simulink model "smm_with_grf_tilting_2d"  (R2014b)
settings: Solver=FixedStepDiscrete  StartTime=0.0  StopTime=inf  FixedStep=sample_time  RelTol=1e-3
undefined symbols (not defined in the file or in its folder): A_kalman_fourbar_gear, A_kalman_transverse, A_kalman_vertical, A_lpf_dtau, A_lpf_leg_spring, alpha_apex, B1_lpf_dtau, B1_lpf_leg_spring, B2_lpf_dtau, B2_lpf_leg_spring, B_kalman_fourbar_gear, B_kalman_transverse, B_kalman_vertical, b_virtual, boom_mount_angle, c_energy, C_kalman_fourbar_gear, C_kalman_transverse, C_kalman_vertical, com_leg_motor, com_torso, contact_threshold, control_start_time, d_vertical_boom_com_offset, d_vertical_com, d_y_com, desired_com_apex_height, desired_com_forward_velocity, desired_torso_angle, Discrete, fcut_contact, g, h_boom, HIP_MTR_MAX_CONT_TORQUE, i_robot, initial_dx_estimate, initial_dy_estimate, initial_dz_estimate, initial_z_estimate, j_leg, j_motor, j_rotor, j_segments, k0_virtual, k_placement, k_sea, kalman_load_to_deflect_transmission, kalman_stance_slip_threshold, kd_lateral, kd_motor, kd_torso, kp_lateral, kp_motor, kp_torso, l0_leg, l0_virtual, l_boom_projected, l_retract_delta, l_retract_swing_max, l_retract_swing_min ... (+59)
libraries: simulink x25, ctrlSharedLib x7, simulink_extras x1
(part 4 of 4)

== matlab function smm_with_grf_tilting_2d/Control/Behavior Control/Lateral Control ==
  data: hopping input; tau_r output size=1; qLateralR input; dqLateralR input; qLateralL input; dqLateralL input; F_leg_R input; F_leg_L input; lateral_transition_force parameter; lateral_target_angle_right parameter; m_leg_motor parameter; m_leg parameter; m_total_real parameter; g parameter; lateral_offset parameter; tau_l output size=1; kp_lateral parameter; kd_lateral parameter; minimum_lateral_angle parameter; maximum_lateral_angle parameter; HIP_MTR_MAX_CONT_TORQUE parameter; torso_centerline_roll_offset_angle parameter
function [tau_r, tau_l] = LateralBoomControl(hopping, qLateralR, dqLateralR, qLateralL, dqLateralL, F_leg_R, F_leg_L, lateral_transition_force, lateral_target_angle_right, m_leg_motor, m_leg, m_total_real, g, lateral_offset, kp_lateral, kd_lateral, minimum_lateral_angle, maximum_lateral_angle, HIP_MTR_MAX_CONT_TORQUE, torso_centerline_roll_offset_angle)
    
    % Only add gravity compensation to PD when suspended from winch (approximately static)
    gravity_compensation = 0;
    if ~hopping, gravity_compensation = (m_leg_motor+m_leg)*g*lateral_offset; end
    
    % Inertia for feedforward accelerations
    motor_inertia = (m_leg_motor+m_leg)*lateral_offset^2;
    
    % Right Leg
    right_target = [lateral_target_angle_right, 0, 0];
    desired = [saturate(right_target(1),minimum_lateral_angle,maximum_lateral_angle), right_target(2)];
    measured = [qLateralR, dqLateralR];
    tau_r = [kp_lateral, kd_lateral] * (desired-measured)' + gravity_compensation + motor_inertia*right_target(3);
    tau_r = max(min(HIP_MTR_MAX_CONT_TORQUE, tau_r),-HIP_MTR_MAX_CONT_TORQUE);
    
    if (F_leg_R >= lateral_transition_force)
        if hopping
            tau_r = -F_leg_R*lateral_offset*(m_total_real-(m_leg_motor+m_leg))/m_total_real;
        else
            tau_r = -lateral_offset*(F_leg_R-(m_leg_motor+m_leg)*g);
        end
    end
    
    % Left Leg
    left_target = [lateral_target_angle_right, 0, 0];
    desired = [saturate(left_target(1),minimum_lateral_angle,maximum_lateral_angle), left_target(2)];
    measured = [qLateralL, dqLateralL];
    tau_l = [kp_lateral, kd_lateral] * (desired-measured)' + gravity_compensation + motor_inertia*left_target(3);
    tau_l = max(min(HIP_MTR_MAX_CONT_TORQUE, tau_l),-HIP_MTR_MAX_CONT_TORQUE);
    
    if (F_leg_L >= lateral_transition_force)
        if hopping
            tau_l = -F_leg_L*lateral_offset*(m_total_real-(m_leg_motor+m_leg))/m_total_real;
        else
            tau_l = -lateral_offset*(F_leg_L-(m_leg_motor+m_leg)*g);
        end
    end
end

function [desired_saturated] = saturate(desired, minimum_lateral_angle, maximum_lateral_angle)
    desired_saturated = desired;
    if desired(1) < minimum_lateral_angle
        desired_saturated = [minimum_lateral_angle, 0];
    elseif desired(1) > maximum_lateral_angle
        desired_saturated = [maximum_lateral_angle, 0];    
    end
end

== matlab function smm_with_grf_tilting_2d/Control/Behavior Control/Torque Distribution Right/Motor Torque Saturation Optimization ==
  data: x1s input; t1 output; x2s input; lambda1 parameter; lambda2 parameter; max_torque_sagittal parameter; t2 output
% Optimal leg motor torque distribution
function [t1, t2] = distribute_torque(x1s, x2s, lambda1, lambda2, max_torque_sagittal)

s = max_torque_sagittal;

% possible solutions
x1 = [                                                      x1s;
                                                            0;
                                                            s;
                                                            0;
                                                           -s;
  (lambda2*s + lambda1*x1s - lambda2*x2s)/(lambda1 + lambda2);
  (lambda1*x1s - lambda2*s + lambda2*x2s)/(lambda1 + lambda2);
  (lambda2*s + lambda1*x1s + lambda2*x2s)/(lambda1 + lambda2);
 -(lambda2*s - lambda1*x1s + lambda2*x2s)/(lambda1 + lambda2)];
 
x2 = [                                                      x2s;
                                                            s;
                                                            0;
                                                           -s;
                                                            0;
  (lambda1*s - lambda1*x1s + lambda2*x2s)/(lambda1 + lambda2);
  (lambda1*s + lambda1*x1s + lambda2*x2s)/(lambda1 + lambda2);
  (lambda1*x1s - lambda1*s + lambda2*x2s)/(lambda1 + lambda2);
 -(lambda1*s + lambda1*x1s - lambda2*x2s)/(lambda1 + lambda2)];

% test constraints
c1 = s - x1 - x2 >= 0;
c2 = s + x1 + x2 >= 0;
c3 = s - x1 + x2 >= 0;
c4 = s + x1 - x2 >= 0;
constraints = c1 & c2 & c3 & c4;

% objective function to maximize
f = -lambda1*(x1-x1s).^2-lambda2*(x2-x2s).^2;
satisfied = find(constraints);
[~,I] = max(f(satisfied));

t1 = x1(satisfied(I));
t2 = x2(satisfied(I));

== matlab function smm_with_grf_tilting_2d/Control/Behavior Control/Primary Leg Behavior/Running/Flight/Calculate Leg Length From Virtual Spring Length ==
  data: phi input; dphi input; l_virtual input; dl_virtual input; pelvis_to_com input; l_leg_target output; d_pelvis_to_com input
function l_leg_target  = VirtualSpringLengthToLegLength2D(phi, dphi, l_virtual, dl_virtual, pelvis_to_com, d_pelvis_to_com)
    [ l_leg_target, ~ ] = VirtualSpringLengthToLegLength2D( phi, dphi, l_virtual, dl_virtual, pelvis_to_com, d_pelvis_to_com );
end

== matlab function smm_with_grf_tilting_2d/Control/Behavior Control/Secondary Leg Behavior/Avoid Hitting Mechanical Limits ==
  data: back_cmd output double; front_cmd output double; dback_cmd output double; dfront_cmd output double; ddback_cmd output double; ddfront_cmd output double; back_desired input; dback_desired input; ddback_desired input; front_desired input; dfront_desired input; ddfront_desired input; min_front_bar_angle parameter; max_front_bar_angle parameter; min_back_bar_angle parameter; max_back_bar_angle parameter
%% Avoid joint limits by ensuring we don't command velocities/accelerations that would push us into them when we are close to them.
function [back_cmd, front_cmd, dback_cmd, dfront_cmd, ddback_cmd, ddfront_cmd] ...
    = AvoidFourbarLimits(back_desired,dback_desired, ddback_desired, ...
          front_desired, dfront_desired, ddfront_desired, ...
          min_front_bar_angle, max_front_bar_angle, min_back_bar_angle, max_back_bar_angle)
    [back_cmd, front_cmd, dback_cmd, dfront_cmd, ddback_cmd, ddfront_cmd] = AvoidFourbarLimits(back_desired,dback_desired, ddback_desired, front_desired, dfront_desired, ddfront_desired, min_front_bar_angle, max_front_bar_angle, min_back_bar_angle, max_back_bar_angle);
end

== matlab function smm_with_grf_tilting_2d/Control/Behavior Control/State Estimation/PositionUsingRobotGeometry ==
  data: right_left input; horizontal_com_position output; roll input; pitch input; yaw input; horizontal_com_velocity output; left_leg_sagittal_angle input; left_leg_lateral_angle input; left_leg_length input; right_leg_sagittal_angle input; right_leg_lateral_angle input; right_leg_length input; m_torso parameter; m_leg_motor parameter; m_leg parameter; com_torso parameter; com_leg_motor parameter; lateral_offset parameter; vertical_com_position output; vertical_com_velocity output; com_left_foot output; dcom_left_foot output; com_right_foot output; dcom_right_foot output; com_pelvis output; dcom_pelvis output
% Returns 2D COM relative to primary foot
function [horizontal_com_position, horizontal_com_velocity, ...
          vertical_com_position, vertical_com_velocity, ...
          com_left_foot, dcom_left_foot, com_right_foot, dcom_right_foot, ....
          com_pelvis, dcom_pelvis] = ...
         ComPositionUsingRobotGeometry(right_left, ...
                                    roll, pitch, yaw, ...
                                    left_leg_sagittal_angle, left_leg_lateral_angle, left_leg_length, ...
                                    right_leg_sagittal_angle, right_leg_lateral_angle, right_leg_length, ...
                                    m_torso, m_leg_motor, m_leg, com_torso, com_leg_motor, lateral_offset)
                    
    q =  [roll(1), pitch(1), yaw(1), left_leg_sagittal_angle(1), left_leg_lateral_angle(1), left_leg_length(1), right_leg_sagittal_angle(1), right_leg_lateral_angle(1), right_leg_length(1)];
    dq = [roll(2), pitch(2), yaw(2), left_leg_sagittal_angle(2), left_leg_lateral_angle(2), left_leg_length(2), right_leg_sagittal_angle(2), right_leg_lateral_angle(2), right_leg_length(2)];
                    
    [ com_pelvis, dcom_pelvis, ...
      com_left_foot, dcom_left_foot, ...
      com_right_foot, dcom_right_foot ] = ...
    ComCalculationFromRobot( q, dq, m_torso, m_leg_motor, m_leg, com_torso, com_leg_motor, lateral_offset );

    if right_left
        com_position = com_right_foot(4:6);
        com_velocity = dcom_right_foot(4:6);
    else
        com_position = com_left_foot(4:6);
        com_velocity = dcom_left_foot(4:6);
    end


    horizontal_com_position = com_position(1);
    horizontal_com_velocity = com_velocity(1);
    vertical_com_position = com_position(3);
    vertical_com_velocity = com_velocity(3);

end

== matlab function smm_with_grf_tilting_2d/Control/Behavior Control/Torque Distribution Left/Motor Torque Saturation Optimization ==
  data: x1s input; t1 output; x2s input; lambda1 parameter; lambda2 parameter; max_torque_sagittal parameter; t2 output
% Optimal leg motor torque distribution
function [t1, t2] = distribute_torque(x1s, x2s, lambda1, lambda2, max_torque_sagittal)

s = max_torque_sagittal;

% possible solutions
x1 = [                                                      x1s;
                                                            0;
                                                            s;
                                                            0;
                                                           -s;
  (lambda2*s + lambda1*x1s - lambda2*x2s)/(lambda1 + lambda2);
  (lambda1*x1s - lambda2*s + lambda2*x2s)/(lambda1 + lambda2);
  (lambda2*s + lambda1*x1s + lambda2*x2s)/(lambda1 + lambda2);
 -(lambda2*s - lambda1*x1s + lambda2*x2s)/(lambda1 + lambda2)];
 
x2 = [                                                      x2s;
                                                            s;
                                                            0;
                                                           -s;
                                                            0;
  (lambda1*s - lambda1*x1s + lambda2*x2s)/(lambda1 + lambda2);
  (lambda1*s + lambda1*x1s + lambda2*x2s)/(lambda1 + lambda2);
  (lambda1*x1s - lambda1*s + lambda2*x2s)/(lambda1 + lambda2);
 -(lambda1*s + lambda1*x1s - lambda2*x2s)/(lambda1 + lambda2)];

% test constraints
c1 = s - x1 - x2 >= 0;
c2 = s + x1 + x2 >= 0;
c3 = s - x1 + x2 >= 0;
c4 = s + x1 - x2 >= 0;
constraints = c1 & c2 & c3 & c4;

% objective function to maximize
f = -lambda1*(x1-x1s).^2-lambda2*(x2-x2s).^2;
satisfied = find(constraints);
[~,I] = max(f(satisfied));

t1 = x1(satisfied(I));
t2 = x2(satisfied(I));

== matlab function smm_with_grf_tilting_2d/Control/Behavior Control/State Estimation/Kalman Filtering/eigen values ==
  data: Z input; E output
function E = eigen(Z)
    E = real(eig(Z));
    E = sort(E);
end

== matlab function smm_with_grf_tilting_2d/Control/Behavior Control/Virtual Spring Calculator/Virtual Spring Calculations ==
  data: th input; alpha_v output; dth input; l input; dl input; phi input; dphi input; dalpha_v output; l_v output; dl_v output; d_vertical_com parameter
function [alpha_v, dalpha_v, l_v, dl_v] = fcn(th, dth, l, dl, phi, dphi, d_vertical_com)

    gma = th + phi;
    dgma = dth + dphi;
    d = d_vertical_com;

    xf  =  l*sin(gma) - d*sin(th);
    dxf =  l*dgma*cos(gma) + dl*sin(gma) - d*dth*cos(th);
    yf  = -l*cos(gma) + d*cos(th);
    dyf =  l*dgma*sin(gma) - dl*cos(gma) - d*dth*sin(th);

    alpha_v  = atan2(yf, xf);
    dalpha_v = 1/(1+(yf/xf)^2) * (xf*dyf - yf*dxf)/xf^2;

    l_v  = (d^2 + l^2 - 2*d*l*cos(phi))^0.5;
    dl_v = (l*dl - d*dl*cos(phi) + d*l*dphi*sin(phi))/l_v;

end

== matlab function smm_with_grf_tilting_2d/Control/Behavior Control/Secondary Leg Behavior/Virtual Leg Trajectory Towards Alpha Apex Target ==
  data: start input; t_system input; l_leg output; dl_leg output; ddl_leg output; phi output; dphi output; ddphi output; alpha_apex parameter; theta input; l_measured input; dl_measured input; phi_measured input; dphi_measured input; d_y_com parameter; l0_virtual parameter
%% Create a trajectory between starting position/velocity and some alpha
% The goal is to move the system towards the alpha target at apex.
function [l_leg, dl_leg, ddl_leg, phi, dphi, ddphi] = fcn(start, t_system, alpha_apex, theta, l_measured, dl_measured, phi_measured, dphi_measured, d_y_com, l0_virtual)
    % Should the target be less than apex position? midpoint?
    [l_apex, dl_apex, ~, phi_apex, dphi_apex, ~] = AlphaTargetToVirtualLeg2D(alpha_apex, 0, 0, theta, 0, 0, d_y_com, l0_virtual);
    
    % Force retraction when secondary leg
    l_apex = 0.8;
    dl_apex = 0;
    
    persistent t_start l_start phi_start dl_start dphi_start;
    if isempty(t_start)
        t_start = t_system;
        l_start = l_measured;
        dl_start = dl_measured;
        phi_start = phi_measured;
        dphi_start = dphi_measured;
    end
    if start %|| (t_system - t_start) > 0.030
        t_start = t_system;
        l_start = l_measured;
        dl_start = dl_measured;
        phi_start = phi_measured;
        dphi_start = dphi_measured;
    end
    

    time_to_takeoff = 0.350;  % Overestimate, How to approximate this?
    t = t_system - t_start;
    t = min(time_to_takeoff, t);
    
    % Virtual Leg Length
    [a0, a1, a2, a3] = ThirdOrderTrajectory(l_start, dl_start, l_apex, dl_apex, time_to_takeoff);
    l_leg = a3*t^3 + a2*t^2 + a1*t + a0;
    dl_leg = 3*a3*t^2 + 2*a2*t + a1;
    ddl_leg = 6*a3*t + 2*a2;
    
    % Virtual Leg Angle
    [a0, a1, a2, a3] = ThirdOrderTrajectory(phi_start, dphi_start, phi_apex, dphi_apex, time_to_takeoff);
    phi = a3*t^3 + a2*t^2 + a1*t + a0;
    dphi = 3*a3*t^2 + 2*a2*t + a1;
    ddphi = 6*a3*t + 2*a2;
end

== matlab function smm_with_grf_tilting_2d/Control/Behavior Control/Secondary Leg Behavior/Virtual Leg to Four Bar ==
  data: l_leg input; dl_leg input; ddl_leg input; phi input; dphi input; ddphi input; back output; dback output; ddback output; front output; dfront output; ddfront output
function [back, dback, ddback, front, dfront, ddfront] = VirtualLegToFourBar(l_leg, dl_leg, ddl_leg, phi, dphi, ddphi)
    [back, dback, ddback, front, dfront, ddfront] = VirtualLegToFourBar(l_leg, dl_leg, ddl_leg, phi, dphi, ddphi);
end

== matlab function smm_with_grf_tilting_2d/Control/Behavior Control/Primary Secondary Leg Swap/ToggleRightLeftLeg ==
  data: toggle input boolean; right_left output double; previous_right_left input double
function right_left = ToggleRightLeftLeg(toggle, previous_right_left)
    
    if toggle
        right_left = -previous_right_left + 1;
    else
        right_left = previous_right_left;
    end

end

== matlab function smm_with_grf_tilting_2d/Control/Behavior Control/Primary Leg Behavior/Running/Stance/Inverse Dynamics Virtual Spring/target_GRF_inverse_dynamics ==
  data: right_left input; z output; k_virtual input; b_virtual input; l_virtual input; theta input; phi input; l_leg input; w input; tau_rotor_f input; tau_rotor_b input; d_vertical_com parameter; l_virtual_rest input; LEG_MTR_GEAR_RATIO parameter; g parameter; j_leg parameter; j_rotor parameter; i_robot parameter; m_total_real parameter; m_leg parameter; GRFx output; GRFy output; kp_torso parameter; kd_torso parameter; desired_torso_angle input; GRF_angle output; max_GRF_angle parameter
%% Inverse dynamics
% Inputs:  gamma, dgamma, theta, dtheta,  GRFx_des, GRFy_des
% Outputs: ddx,   ddy,    ddl,   ddgamma, ddtheta,  tau_sf,  tau_sb
function [z, GRFx, GRFy, GRF_angle]  = fcn(right_left, k_virtual, b_virtual, l_virtual, theta, phi, l_leg, w,...
                  tau_rotor_f, tau_rotor_b, ...
                  d_vertical_com, l_virtual_rest, LEG_MTR_GEAR_RATIO, g,...
                  j_leg, j_rotor, i_robot, ...
                  m_total_real, m_leg, ...
                  kp_torso, kd_torso, desired_torso_angle, max_GRF_angle)

              
              
    % Parameters
    m      = m_total_real;      % mass of system + boom
    Il     = j_leg;             % inertia of leg
    Ir     = j_rotor;           % inertia of rotor
    It     = i_robot;           % inertia of system.
    d      = d_vertical_com;    % distance from hip to system COM
    g1     = phi(1)+theta(1);   % global leg angle (after spring)
    dg1    = phi(2)+theta(2);
    th     = theta(1);          % global torso angle   
    dth    = theta(2);
    t_rf   = tau_rotor_f;       % torque applied at front rotor 
    t_rb   = tau_rotor_b;       % torque applied at back rotor
    N      = -LEG_MTR_GEAR_RATIO;
    l      = l_leg(1);          % leg length
    dl     = l_leg(2);
    lv     = l_virtual(1);      % virtual spring length
    dlv = l_virtual(2);
    dx     = -l*dg1*cos(g1)+dth*cos(th);
    dy     = l*dg1*sin(g1)-dth*sin(th);
    
    
    
    % Target GRFs
    delta_lv = l_virtual_rest -  lv;
    F_virtual = k_virtual*delta_lv + b_virtual*dlv;
    GRF = F_virtual* ...
                        [(d*sin(th)-l*sin(g1))/lv; ...
                         (d*cos(th)-l*cos(g1))/lv];
    GRF_angle = atan2(GRF(2),GRF(1));
                     
                     
                     
    % Trunk posture correction 
    % l_leg cross GRF = I_robot * ddtheta
    F_reg = 1; % prevent division by zero
    ddth_desired = kp_torso*(desired_torso_angle - th) - kd_torso*dth; % PD law
    sine_ratio = It*ddth_desired / (lv*(norm(GRF) + F_reg));
    max_angle = 20*pi/180;
    sine_ratio = min(sin(max_angle), max(-sin(max_angle), sine_ratio));  % saturate rotation angle
    GRF_rotation = asin(sine_ratio);
    GRF_full_angle = GRF_rotation + GRF_angle; % saturate GRF angle
    if GRF_full_angle > (pi-max_GRF_angle)
        GRF_rotation = (pi-max_GRF_angle) - GRF_angle;
    elseif GRF_full_angle < max_GRF_angle
        GRF_rotation = max_GRF_angle - GRF_angle;  
    end
    R = [cos(GRF_rotation)  -sin(GRF_rotation); sin(GRF_rotation) cos(GRF_rotation)];
    GRF_target = R*GRF; % rotate GRF CCW
    GRFx = GRF_target(1);
    GRFy = GRF_target(2);
    GRF_angle = atan2(GRFy,GRFx);
    
%     % Boom assymetry compensation
%     if right_left 
%         GRFy = (1.97/1.75)*GRFy;
%     end
%     
    % Stance dynamics (P z = [h; -dJ*dq] + [J zeros(2,2)]^T F)
    %     J  = [1  0  sin(g1)     l*cos(g1)   -d*cos(th);
    %           0  1  cos(g1)    -l*sin(g1)    d*sin(th)];
    %       
    %     dJ = [0  0   dg1*cos(g1)    (-l*dg1*sin(g1)+dl*cos(g1))  d*dth*sin(th);
    %           0  0  -dg1*sin(g1)    (-1*dg1*cos(g1)-dl*sin(g1))  d*dth*cos(th)];
    % 
    %     dq  = [dx  dy  dl  dg1  dth ]';
    %       
    %     M = [m  0   0       0    0; 
    %          0  m   0       0    0;
    %          0  0   m_leg   0    0;   
    %          0  0   0       Il   0;  
    %          0  0   0       0    It];  
    %     
    %     h = [0; -m*g_reduced; 0; 0; (-t_rf-t_rb)];
    % 
    %     S = [ 0         0;
    %           0         0;
    %           1/w      -1/w;
    %           1         1;
    %          -(N-1)/N  -(N-1)/N];
    % 
    %     F = [GRFx GRFy]';
    %     
    %     P = [M              -S;       
    %          J               zeros(2,2)];
    
    % Solving for z:    
    %     ddq = [ddx ddy ddl ddg1 ddth]';
    %     z = [ddq; t_sf; t_sb];
    %     z = P\([h; -dJ*dq] + [J zeros(2,2)]'*F);
    
    z =  [GRFx/m;
         (GRFy - g*m)/m;
        -(Il*d*dg1^2*m*cos(g1 - th) - 2*GRFx*Il*d*sin(th) - 2*Il*d^2*dth^2*m - GRFy*d*l^2*m*cos(th) - GRFx*d*l^2*m*sin(th) - 2*GRFy*Il*d*cos(th) + 2*GRFy*It*N*l*cos(g1) + 2*GRFy*Il*N*d*cos(th) + 2*GRFx*It*N*l*sin(g1) + 2*GRFx*Il*N*d*sin(th) - It*N*dg1^2*l*m + GRFy*d*l^2*m*cos(2*g1 - th) + GRFx*d*l^2*m*sin(2*g1 - th) + 2*Il*d*g*m*cos(th) + Il*d*dg1^2*m*cos(g1 + th) + 2*Il*N*d^2*dth^2*m - It*N*dg1^2*l^2*m - 2*It*N*g*l*m*cos(g1) - 2*Il*N*d*g*m*cos(th) + It*N*dg1^2*l^2*m*cos(2*g1) - Il*N*d*dg1^2*m*cos(g1 + th) - Il*d*dg1^2*l*m*cos(g1 + th) + 4*Il*d*dg1*dl*m*sin(g1 - th) + GRFy*N*d^2*l*m*cos(g1) + GRFy*N*d*l^2*m*cos(th) + GRFx*N*d^2*l*m*sin(g1) + 2*N*d*l*m*t_rb*sin(g1 - th) + 2*N*d*l*m*t_rf*sin(g1 - th) + GRFx*N*d*l^2*m*sin(th) - Il*N*d*dg1^2*m*cos(g1 - th) - GRFy*N*d^2*l*m*cos(g1 - 2*th) + GRFx*N*d^2*l*m*sin(g1 - 2*th) + Il*d*dg1^2*l*m*cos(g1 - th) - It*N*dg1^2*l*m*cos(2*g1) - GRFy*N*d*l^2*m*cos(2*g1 - th) - GRFx*N*d*l^2*m*sin(2*g1 - th) + Il*N*d*dg1^2*l*m*cos(g1 + th) - 4*Il*N*d*dg1*dl*m*sin(g1 - th) - Il*N*d*dg1^2*l*m*cos(g1 - th) + 2*It*N*d*dth^2*l*m*cos(g1 - th))/(2*m*(It*N*l - Il*d*cos(g1 - th) + Il*N*d*cos(g1 - th)));
        -(2*GRFx*It*N*cos(g1) - 2*GRFy*It*N*sin(g1) + GRFx*N*d^2*m*cos(g1 - 2*th) + 4*It*N*dg1*dl*m + GRFy*N*d^2*m*sin(g1 - 2*th) + GRFx*d*l*m*cos(2*g1 - th) - GRFy*d*l*m*sin(2*g1 - th) + It*N*dg1^2*m*sin(2*g1) + 2*It*N*g*m*sin(g1) + GRFx*d*l*m*cos(th) - GRFy*d*l*m*sin(th) + GRFx*N*d^2*m*cos(g1) + 2*N*d*m*t_rb*cos(g1 - th) + 2*N*d*m*t_rf*cos(g1 - th) - GRFy*N*d^2*m*sin(g1) - GRFx*N*d*l*m*cos(th) + GRFy*N*d*l*m*sin(th) - GRFx*N*d*l*m*cos(2*g1 - th) - 2*It*N*d*dth^2*m*sin(g1 - th) + GRFy*N*d*l*m*sin(2*g1 - th) - It*N*dg1^2*l*m*sin(2*g1))/(2*m*(It*N*l - Il*d*cos(g1 - th) + Il*N*d*cos(g1 - th)));
        -(GRFx*Il*cos(g1) - GRFy*Il*sin(g1) - GRFx*Il*N*cos(g1) + (Il*dg1^2*m*sin(2*g1))/2 + GRFy*Il*N*sin(g1) + Il*g*m*sin(g1) + GRFx*l^2*m*cos(g1) - GRFy*l^2*m*sin(g1) + 2*Il*dg1*dl*m + N*l*m*t_rb + N*l*m*t_rf + GRFy*N*l^2*m*sin(g1) - 2*Il*N*dg1*dl*m - Il*d*dth^2*m*sin(g1 - th) - (Il*N*dg1^2*m*sin(2*g1))/2 - (Il*dg1^2*l*m*sin(2*g1))/2 - Il*N*g*m*sin(g1) - GRFx*N*l^2*m*cos(g1) + GRFx*N*d*l*m*cos(th) - GRFy*N*d*l*m*sin(th) + Il*N*d*dth^2*m*sin(g1 - th) + (Il*N*dg1^2*l*m*sin(2*g1))/2)/(m*(It*N*l - Il*d*cos(g1 - th) + Il*N*d*cos(g1 - th)));
        -(2*GRFx*Il*It*N*cos(g1) - 2*GRFy*Il*It*N*sin(g1) - GRFy*Il*d*m*w*cos(th) - 2*GRFy*Il*d*m_leg*w*cos(th) - GRFx*Il*d*m*w*sin(th) - 2*GRFx*Il*d*m_leg*w*sin(th) + GRFx*Il*N*d^2*m*cos(g1) + 2*Il*N*d*m*t_rb*cos(g1 - th) + 2*Il*N*d*m*t_rf*cos(g1 - th) + 2*GRFx*It*N*l^2*m*cos(g1) - GRFy*Il*N*d^2*m*sin(g1) - 2*GRFy*It*N*l^2*m*sin(g1) + GRFx*Il*N*d^2*m*cos(g1 - 2*th) + 4*Il*It*N*dg1*dl*m + GRFy*Il*N*d^2*m*sin(g1 - 2*th) - 2*Il*d^2*dth^2*m*m_leg*w - GRFy*Il*d*m*w*cos(2*g1 - th) - GRFx*Il*d*m*w*sin(2*g1 - th) + Il*It*N*dg1^2*m*sin(2*g1) + 2*Il*It*N*g*m*sin(g1) - GRFx*d*l^2*m*m_leg*w*sin(th) - Il*It*N*dg1^2*l*m*sin(2*g1) + Il*d*dg1^2*m*m_leg*w*cos(g1 - th) + 2*GRFy*It*N*l*m*w*cos(g1) + 2*GRFy*It*N*l*m_leg*w*cos(g1) + GRFy*Il*N*d*m*w*cos(th) + 2*GRFy*Il*N*d*m_leg*w*cos(th) + 2*GRFx*It*N*l*m*w*sin(g1) + 2*GRFx*It*N*l*m_leg*w*sin(g1) + GRFx*Il*N*d*m*w*sin(th) + 2*GRFx*Il*N*d*m_leg*w*sin(th) - It*N*dg1^2*l*m*m_leg*w + GRFy*d*l^2*m*m_leg*w*cos(2*g1 - th) + GRFx*d*l^2*m*m_leg*w*sin(2*g1 - th) + 2*Il*d*g*m*m_leg*w*cos(th) + Il*d*dg1^2*m*m_leg*w*cos(g1 + th) + 2*Il*N*d^2*dth^2*m*m_leg*w - It*N*dg1^2*l^2*m*m_leg*w - 2*Il*It*N*d*dth^2*m*sin(g1 - th) + GRFy*Il*N*d*m*w*cos(2*g1 - th) + GRFx*Il*N*d*m*w*sin(2*g1 - th) - GRFy*d*l^2*m*m_leg*w*cos(th) + It*N*dg1^2*l^2*m*m_leg*w*cos(2*g1) - Il*N*d*dg1^2*m*m_leg*w*cos(g1 + th) - Il*d*dg1^2*l*m*m_leg*w*cos(g1 + th) + 4*Il*d*dg1*dl*m*m_leg*w*sin(g1 - th) + GRFy*N*d^2*l*m*m_leg*w*cos(g1) + GRFy*N*d*l^2*m*m_leg*w*cos(th) + GRFx*N*d^2*l*m*m_leg*w*sin(g1) + 2*N*d*l*m*m_leg*t_rb*w*sin(g1 - th) + 2*N*d*l*m*m_leg*t_rf*w*sin(g1 - th) + GRFx*N*d*l^2*m*m_leg*w*sin(th) - Il*N*d*dg1^2*m*m_leg*w*cos(g1 - th) - GRFy*N*d^2*l*m*m_leg*w*cos(g1 - 2*th) + GRFx*N*d^2*l*m*m_leg*w*sin(g1 - 2*th) + Il*d*dg1^2*l*m*m_leg*w*cos(g1 - th) - It*N*dg1^2*l*m*m_leg*w*cos(2*g1) - GRFy*N*d*l^2*m*m_leg*w*cos(2*g1 - th) - GRFx*N*d*l^2*m*m_leg*w*sin(2*g1 - th) - 2*It*N*g*l*m*m_leg*w*cos(g1) - 2*Il*N*d*g*m*m_leg*w*cos(th) + Il*N*d*dg1^2*l*m*m_leg*w*cos(g1 + th) - 4*Il*N*d*dg1*dl*m*m_leg*w*sin(g1 - th) - Il*N*d*dg1^2*l*m*m_leg*w*cos(g1 - th) + 2*It*N*d*dth^2*l*m*m_leg*w*cos(g1 - th))/(4*m*(It*N*l - Il*d*cos(g1 - th) + Il*N*d*cos(g1 - th)));
         (2*GRFy*Il*It*N*sin(g1) - 2*GRFx*Il*It*N*cos(g1) - GRFy*Il*d*m*w*cos(th) - 2*GRFy*Il*d*m_leg*w*cos(th) - GRFx*Il*d*m*w*sin(th) - 2*GRFx*Il*d*m_leg*w*sin(th) - GRFx*Il*N*d^2*m*cos(g1) - 2*Il*N*d*m*t_rb*cos(g1 - th) - 2*Il*N*d*m*t_rf*cos(g1 - th) - 2*GRFx*It*N*l^2*m*cos(g1) + GRFy*Il*N*d^2*m*sin(g1) + 2*GRFy*It*N*l^2*m*sin(g1) - GRFx*Il*N*d^2*m*cos(g1 - 2*th) - 4*Il*It*N*dg1*dl*m - GRFy*Il*N*d^2*m*sin(g1 - 2*th) - 2*Il*d^2*dth^2*m*m_leg*w - GRFy*Il*d*m*w*cos(2*g1 - th) - GRFx*Il*d*m*w*sin(2*g1 - th) - Il*It*N*dg1^2*m*sin(2*g1) - 2*Il*It*N*g*m*sin(g1) - GRFx*d*l^2*m*m_leg*w*sin(th) + Il*It*N*dg1^2*l*m*sin(2*g1) + Il*d*dg1^2*m*m_leg*w*cos(g1 - th) + 2*GRFy*It*N*l*m*w*cos(g1) + 2*GRFy*It*N*l*m_leg*w*cos(g1) + GRFy*Il*N*d*m*w*cos(th) + 2*GRFy*Il*N*d*m_leg*w*cos(th) + 2*GRFx*It*N*l*m*w*sin(g1) + 2*GRFx*It*N*l*m_leg*w*sin(g1) + GRFx*Il*N*d*m*w*sin(th) + 2*GRFx*Il*N*d*m_leg*w*sin(th) - It*N*dg1^2*l*m*m_leg*w + GRFy*d*l^2*m*m_leg*w*cos(2*g1 - th) + GRFx*d*l^2*m*m_leg*w*sin(2*g1 - th) + 2*Il*d*g*m*m_leg*w*cos(th) + Il*d*dg1^2*m*m_leg*w*cos(g1 + th) + 2*Il*N*d^2*dth^2*m*m_leg*w - It*N*dg1^2*l^2*m*m_leg*w + 2*Il*It*N*d*dth^2*m*sin(g1 - th) + GRFy*Il*N*d*m*w*cos(2*g1 - th) + GRFx*Il*N*d*m*w*sin(2*g1 - th) - GRFy*d*l^2*m*m_leg*w*cos(th) + It*N*dg1^2*l^2*m*m_leg*w*cos(2*g1) - Il*N*d*dg1^2*m*m_leg*w*cos(g1 + th) - Il*d*dg1^2*l*m*m_leg*w*cos(g1 + th) + 4*Il*d*dg1*dl*m*m_leg*w*sin(g1 - th) + GRFy*N*d^2*l*m*m_leg*w*cos(g1) + GRFy*N*d*l^2*m*m_leg*w*cos(th) + GRFx*N*d^2*l*m*m_leg*w*sin(g1) + 2*N*d*l*m*m_leg*t_rb*w*sin(g1 - th) + 2*N*d*l*m*m_leg*t_rf*w*sin(g1 - th) + GRFx*N*d*l^2*m*m_leg*w*sin(th) - Il*N*d*dg1^2*m*m_leg*w*cos(g1 - th) - GRFy*N*d^2*l*m*m_leg*w*cos(g1 - 2*th) + GRFx*N*d^2*l*m*m_leg*w*sin(g1 - 2*th) + Il*d*dg1^2*l*m*m_leg*w*cos(g1 - th) - It*N*dg1^2*l*m*m_leg*w*cos(2*g1) - GRFy*N*d*l^2*m*m_leg*w*cos(2*g1 - th) - GRFx*N*d*l^2*m*m_leg*w*sin(2*g1 - th) - 2*It*N*g*l*m*m_leg*w*cos(g1) - 2*Il*N*d*g*m*m_leg*w*cos(th) + Il*N*d*dg1^2*l*m*m_leg*w*cos(g1 + th) - 4*Il*N*d*dg1*dl*m*m_leg*w*sin(g1 - th) - Il*N*d*dg1^2*l*m*m_leg*w*cos(g1 - th) + 2*It*N*d*dth^2*l*m*m_leg*w*cos(g1 - th))/(4*m*(It*N*l - Il*d*cos(g1 - th) + Il*N*d*cos(g1 - th)))];


end

== matlab function smm_with_grf_tilting_2d/Control/Behavior Control/Primary Leg Behavior/Running/Flight/Avoid Hitting Mechanical Limits ==
  data: back_cmd output double; front_cmd output double; dback_cmd output double; dfront_cmd output double; ddback_cmd output double; ddfront_cmd output double; back_desired input; dback_desired input; ddback_desired input; front_desired input; dfront_desired input; ddfront_desired input; min_front_bar_angle parameter; max_front_bar_angle parameter; min_back_bar_angle parameter; max_back_bar_angle parameter
%% Avoid joint limits by ensuring we don't command velocities/accelerations that would push us into them when we are close to them.
function [back_cmd, front_cmd, dback_cmd, dfront_cmd, ddback_cmd, ddfront_cmd] ...
    = AvoidFourbarLimits(back_desired,dback_desired, ddback_desired, ...
          front_desired, dfront_desired, ddfront_desired, ...
          min_front_bar_angle, max_front_bar_angle, min_back_bar_angle, max_back_bar_angle)
    [back_cmd, front_cmd, dback_cmd, dfront_cmd, ddback_cmd, ddfront_cmd] = AvoidFourbarLimits(back_desired,dback_desired, ddback_desired, front_desired, dfront_desired, ddfront_desired, min_front_bar_angle, max_front_bar_angle, min_back_bar_angle, max_back_bar_angle);
end

== matlab function smm_with_grf_tilting_2d/Control/Behavior Control/Primary Leg Behavior/Running/Flight/Virtual Leg to Four Bar ==
  data: l_leg input; dl_leg input; ddl_leg input; phi input; dphi input; ddphi input; back output; dback output; ddback output; front output; dfront output; ddfront output
function [back, dback, ddback, front, dfront, ddfront] = VirtualLegToFourBar(l_leg, dl_leg, ddl_leg, phi, dphi, ddphi)
    [back, dback, ddback, front, dfront, ddfront] = VirtualLegToFourBar(l_leg, dl_leg, ddl_leg, phi, dphi, ddphi);
end

== matlab function smm_with_grf_tilting_2d/Control/Behavior Control/Primary Leg Behavior/Running/Flight/Leg Extension Trajectory1 ==
  data: back input; front input; l_leg output double
function l_leg  = LegLengthCalculator(back, front)
    l_leg = cos((back-front)/2);
end

== matlab function smm_with_grf_tilting_2d/Control/Behavior Control/Primary Leg Behavior/Running/Flight/Leg Extension Trajectory ==
  data: t input double; t_trajectory input double; l_leg_final input double; l_leg_initial input double; l_leg output double; dl_leg output double; ddl_leg output double; max_leg_velocity parameter; max_leg_acceleration parameter; min_leg_extension_time parameter
function [l_leg, dl_leg, ddl_leg] = LegLengthTrajectory(t, t_trajectory, l_leg_final, l_leg_initial, max_leg_velocity, max_leg_acceleration, min_leg_extension_time)
    t_trajectory = max(min_leg_extension_time, t_trajectory);
    [l_leg, dl_leg, ddl_leg] = LegLengthTrajectory(t, l_leg_initial, l_leg_final, t_trajectory, max_leg_velocity, max_leg_acceleration);
end

== matlab function smm_with_grf_tilting_2d/Control/Behavior Control/Secondary Leg Behavior/Mirrored Leg Length Target ==
  data: primary_l_leg input; l_leg output; dl_leg output; primary_dl_leg input; l_retract_swing_min parameter; l_retract_swing_max parameter; ddl_leg output; l_retract_delta parameter
function [l_leg, dl_leg, ddl_leg] = LegLengthTarget(primary_l_leg, primary_dl_leg, l_retract_swing_min, l_retract_swing_max, l_retract_delta)

    l_leg = primary_l_leg - l_retract_delta;
    dl_leg = 0;
    ddl_leg = 0;
    if l_leg > l_retract_swing_min && l_leg < l_retract_swing_max
        dl_leg = primary_dl_leg;
    else
        l_leg = max(min(l_leg, l_retract_swing_max), l_retract_swing_min);
    end

end

== matlab function smm_with_grf_tilting_2d/Control/Behavior Control/Primary Leg Behavior/Running/Flight/TogglePositiveNegative ==
  data: toggle input boolean; output output double; previous input double
function output = Toggle(toggle, previous)
    
    if toggle
        output = -previous;
    else
        output = previous;
    end

end

== matlab function smm_with_grf_tilting_2d/Control/Behavior Control/State Estimation/PositionUsingBoomEncoders ==
  data: horizontal_com_position output; qRoll input; dqRoll input; qYaw input; horizontal_com_velocity output; vertical_com_position output; dqYaw input; qPitch input; dqPitch input; l_boom_projected parameter; h_boom parameter; boom_mount_angle parameter; d_vertical_boom_com_offset parameter; vertical_com_velocity output
function [horizontal_com_position, horizontal_com_velocity, ...
          vertical_com_position, vertical_com_velocity] = ...
         PositionUsingBoomEncoders(qRoll, dqRoll, qYaw, dqYaw, qPitch, dqPitch, ...
                        l_boom_projected, h_boom, boom_mount_angle, ...
                        d_vertical_boom_com_offset)
    
    % com position / velocity
    [ horizontal_com_position, horizontal_com_velocity, vertical_com_position, vertical_com_velocity, ~, ~ ] = ComCalculationFromBoom( qRoll, dqRoll, qYaw, dqYaw, qPitch, dqPitch, l_boom_projected, h_boom, boom_mount_angle, d_vertical_boom_com_offset );
    
end

== matlab function smm_with_grf_tilting_2d/Fourbar Gearside Kalman Filter/External Trunk Torque Estimate ==
  data: grf_xz input; rotor_torque input; spring_torque input; tau_trunk output; torso_pitch input; d_vertical_com parameter; LEG_MTR_GEAR_RATIO parameter
function tau_trunk = tau_trunk(grf_xz, rotor_torque, spring_torque, torso_pitch, d_vertical_com, LEG_MTR_GEAR_RATIO )
    d = d_vertical_com;
    theta = torso_pitch;
    N = LEG_MTR_GEAR_RATIO;
    tau_trunk = sum(-rotor_torque + -(N-1)/N*spring_torque) + (-d*cos(theta)*grf_xz(1) + d*sin(theta)*grf_xz(2));
end

== matlab function smm_with_grf_tilting_2d/Fourbar Gearside Kalman Filter/Covariance Estimates ==
  data: spring_torque input; absolute_gear input; current_position_estimate input; state_uncertainty input; Q1 output; R1 output; Q2 output; R2 output; R_kalman_absolute_normal parameter; R_kalman_absolute_fail parameter; R_kalman_incremental_unloaded parameter; R_kalman_incremental_loaded parameter; kalman_load_to_deflect_transmission parameter; Q3 output; R3 output; Q4 output; R4 output; max_absolute_measurement_innovation parameter; k_sea parameter; Q_kalman_spring_torque parameter; Q_kalman_rotor_torque parameter; Q_kalman_trunk_torque parameter; sample_time parameter
function [Q1, R1, Q2, R2, Q3, R3, Q4, R4] = covariance( spring_torque, absolute_gear, current_position_estimate, state_uncertainty, R_kalman_absolute_normal, R_kalman_absolute_fail, R_kalman_incremental_unloaded, R_kalman_incremental_loaded, kalman_load_to_deflect_transmission, max_absolute_measurement_innovation, k_sea, Q_kalman_spring_torque, Q_kalman_rotor_torque, Q_kalman_trunk_torque, sample_time)

    persistent previous_absolute_gear
    if isempty(previous_absolute_gear)
        previous_absolute_gear = absolute_gear;
    end
    
    % Measurement covariance
    R_absolute = ones(4,1)*R_kalman_absolute_normal;
    dropped_out = previous_absolute_gear == absolute_gear;
    out_of_range = abs(current_position_estimate - absolute_gear) > max_absolute_measurement_innovation;
    R_absolute(dropped_out | out_of_range) = R_kalman_absolute_fail;
    
    R_incremental_scale = min(abs(spring_torque)/kalman_load_to_deflect_transmission, 1);
    R_incremental = R_incremental_scale*R_kalman_incremental_loaded + (1-R_incremental_scale)*R_kalman_incremental_unloaded;
    
    R1 = diag([R_absolute(1), R_incremental(1)])/sample_time;
    R2 = diag([R_absolute(2), R_incremental(2)])/sample_time;
    R3 = diag([R_absolute(3), R_incremental(3)])/sample_time;
    R4 = diag([R_absolute(4), R_incremental(4)])/sample_time;
    
    % Process noise covariance
    Q_spring_torque = k_sea'.^2.*(state_uncertainty + R_kalman_absolute_normal) + Q_kalman_spring_torque;

    Q1 = diag([Q_spring_torque(1), Q_kalman_rotor_torque, Q_kalman_trunk_torque]);
    Q2 = diag([Q_spring_torque(2), Q_kalman_rotor_torque, Q_kalman_trunk_torque]);
    Q3 = diag([Q_spring_torque(3), Q_kalman_rotor_torque, Q_kalman_trunk_torque]);
    Q4 = diag([Q_spring_torque(4), Q_kalman_rotor_torque, Q_kalman_trunk_torque]);

    previous_absolute_gear = absolute_gear;
end

== matlab function smm_with_grf_tilting_2d/Fourbar Gearside Kalman Filter/eigen values 1 ==
  data: Z input; E output
function E = eigen(Z)
    E = real(eig(Z));
    E = sort(E);
end

== matlab function smm_with_grf_tilting_2d/Fourbar Gearside Kalman Filter/eigen values 2 ==
  data: Z input; E output
function E = eigen(Z)
    E = real(eig(Z));
    E = sort(E);
end

== matlab function smm_with_grf_tilting_2d/Fourbar Gearside Kalman Filter/eigen values 3 ==
  data: Z input; E output
function E = eigen(Z)
    E = real(eig(Z));
    E = sort(E);
end

== matlab function smm_with_grf_tilting_2d/Fourbar Gearside Kalman Filter/eigen values4  ==
  data: Z input; E output
function E = eigen(Z)
    E = real(eig(Z));
    E = sort(E);
end

== matlab function smm_with_grf_tilting_2d/Control/Behavior Control/Primary Leg Behavior/Running/Flight/Deadbeat Placement/Avoid Hitting Mechanical Limits1 ==
  data: back_cmd output; front_cmd output; dback_cmd output; dfront_cmd output; ddback_cmd output; ddfront_cmd output; back_desired input; dback_desired input; ddback_desired input; front_desired input; dfront_desired input; ddfront_desired input; min_front_bar_angle parameter; max_front_bar_angle parameter; min_back_bar_angle parameter; max_back_bar_angle parameter
%% Avoid joint limits by ensuring we don't command velocities/accelerations that would push us into them when we are close to them.
function [back_cmd, front_cmd, dback_cmd, dfront_cmd, ddback_cmd, ddfront_cmd] ...
    = AvoidFourbarLimits(back_desired,dback_desired, ddback_desired, ...
          front_desired, dfront_desired, ddfront_desired, ...
          min_front_bar_angle, max_front_bar_angle, min_back_bar_angle, max_back_bar_angle)
    [back_cmd, front_cmd, dback_cmd, dfront_cmd, ddback_cmd, ddfront_cmd] = AvoidFourbarLimits(back_desired,dback_desired, ddback_desired, front_desired, dfront_desired, ddfront_desired, min_front_bar_angle, max_front_bar_angle, min_back_bar_angle, max_back_bar_angle);
end

== matlab function smm_with_grf_tilting_2d/Control/Behavior Control/Primary Leg Behavior/Running/Flight/Deadbeat Placement/Leg Trajectory Generator (Level Ground)/Alpha Target to Leg Length and Leg Angle ==
  data: alpha_v input; dalpha_v input; ddalpha_v input; theta input; dtheta input; l output; dl output; ddl output; phi output; d_y_com parameter; l0_virtual parameter; dphi output; ddphi output
function [l, dl, ddl, phi, dphi, ddphi] = fcn(alpha_v, dalpha_v, ddalpha_v, theta, dtheta, d_y_com, l0_virtual)
    [l, dl, ddl, phi, dphi, ddphi] = AlphaTargetToVirtualLeg2D(alpha_v, dalpha_v, ddalpha_v, theta, dtheta, 0, d_y_com, l0_virtual);
end

== matlab function smm_with_grf_tilting_2d/Control/Behavior Control/Primary Leg Behavior/Running/Flight/Deadbeat Placement/Leg Trajectory Generator (Level Ground)/Retracted Leg Trajectory ==
  data: start input; t_system input; t_apex input; l_apex input; dl_apex input; phi_apex input; dphi_apex input; l_measured input; dl_measured input; phi_measured input; l output; dl output; ddl output; phi output; dphi output; ddphi output; dphi_measured input
%% Generates a dynamically feasible trajectory for swinging the virtual leg between two points.
% Constrains to starting/ending positions and velocities.
% Minimizes torque squared
% May want to generate the trajectory in fourbar coordinates instead.
function [l, dl, ddl, phi, dphi, ddphi] = fcn(start, t_system, t_apex, l_apex, dl_apex, phi_apex, dphi_apex, l_measured, dl_measured, phi_measured, dphi_measured)

    persistent t_start l_start phi_start dl_start dphi_start;
    if isempty(t_start) || start
        t_start = t_system;
        l_start = l_measured;
        dl_start = dl_measured;
        phi_start = phi_measured;
        dphi_start = dphi_measured;
    end
    
    t = t_system - t_start;
    time_to_apex = 0.95*2*(t_apex - t_start);
    t = min(time_to_apex, t);

    % Virtual Leg Length
    [a0, a1, a2, a3] = ThirdOrderTrajectory(l_start, dl_start, l_apex, dl_apex, time_to_apex);
    l = a3*t^3 + a2*t^2 + a1*t + a0;
    dl = 3*a3*t^2 + 2*a2*t + a1;
    ddl = 6*a3*t + 2*a2;
    
    % Virtual Leg Angle
    [a0, a1, a2, a3] = ThirdOrderTrajectory(phi_start, dphi_start, phi_apex, dphi_apex, time_to_apex);
    phi = a3*t^3 + a2*t^2 + a1*t + a0;
    dphi = 3*a3*t^2 + 2*a2*t + a1;
    ddphi = 6*a3*t + 2*a2;

end

== matlab function smm_with_grf_tilting_2d/Control/Behavior Control/Primary Leg Behavior/Running/Flight/Deadbeat Placement/Leg Trajectory Generator (Normal)/Alpha Target to Leg Length and Leg Angle ==
  data: alpha_v input; dalpha_v input; ddalpha_v input; theta input; dtheta input; l output; dl output; ddl output; phi output; d_y_com parameter; l0_virtual parameter; dphi output; ddphi output
function [l, dl, ddl, phi, dphi, ddphi] = fcn(alpha_v, dalpha_v, ddalpha_v, theta, dtheta, d_y_com, l0_virtual)
    [l, dl, ddl, phi, dphi, ddphi] = AlphaTargetToVirtualLeg2D(alpha_v, dalpha_v, ddalpha_v, theta, dtheta, 0, d_y_com, l0_virtual);
end

== matlab function smm_with_grf_tilting_2d/Control/Behavior Control/Primary Leg Behavior/Running/Flight/Deadbeat Placement/Leg Trajectory Generator (Normal)/Avoid Virtual Leg Length Limits ==
  data: l_leg_desired input; dl_leg_desired input; ddl_leg_desired input; l_leg_cmd output double; dl_leg_cmd output double; ddl_leg_cmd output double; min_leg_length parameter; max_leg_length parameter
%% Avoid virtual leg length limits by ensuring we don't command position/velocities/accelerations that would hit them.
function [l_leg_cmd, dl_leg_cmd, ddl_leg_cmd] = AvoidVirtualLengthLimits(l_leg_desired, dl_leg_desired, ddl_leg_desired, min_leg_length, max_leg_length)
    [l_leg_cmd, dl_leg_cmd, ddl_leg_cmd] = AvoidVirtualLengthLimits(l_leg_desired, dl_leg_desired, ddl_leg_desired, min_leg_length, max_leg_length);
end

== matlab function smm_with_grf_tilting_2d/Control/Behavior Control/Primary Leg Behavior/Running/Flight/Deadbeat Placement/Leg Trajectory Generator (Normal)/Avoid Virtual Leg Length Limits1 ==
  data: l_leg_desired input; dl_leg_desired input; ddl_leg_desired input; l_leg_cmd output double; dl_leg_cmd output double; ddl_leg_cmd output double; min_leg_length parameter; max_leg_length parameter
%% Avoid virtual leg length limits by ensuring we don't command position/velocities/accelerations that would hit them.
function [l_leg_cmd, dl_leg_cmd, ddl_leg_cmd] = AvoidVirtualLengthLimits(l_leg_desired, dl_leg_desired, ddl_leg_desired, min_leg_length, max_leg_length)
    [l_leg_cmd, dl_leg_cmd, ddl_leg_cmd] = AvoidVirtualLengthLimits(l_leg_desired, dl_leg_desired, ddl_leg_desired, min_leg_length, max_leg_length);
end

== matlab function smm_with_grf_tilting_2d/Control/Behavior Control/Primary Leg Behavior/Running/Flight/Deadbeat Placement/Leg Trajectory Generator (Normal)/Retracted Leg Trajectory ==
  data: start input boolean; t_system input double; t_apex input double; l_apex input double; dl_apex input double; phi_apex input double; dphi_apex input double; l_measured input double; dl_measured input double; phi_measured input double; l output double; dl output double; ddl output double; phi output double; dphi output double; ddphi output double; dphi_measured input double
%% Generates a dynamically feasible trajectory for swinging the virtual leg between two points.
% Constrains to starting/ending positions and velocities.
% Minimizes torque squared
% May want to generate the trajectory in fourbar coordinates instead.
function [l, dl, ddl, phi, dphi, ddphi] = fcn(start, t_system, t_apex, l_apex, dl_apex, phi_apex, dphi_apex, l_measured, dl_measured, phi_measured, dphi_measured)

    persistent t_start l_start phi_start dl_start dphi_start;
    if isempty(t_start)
        t_start = t_system;
        l_start = l_measured;
        dl_start = dl_measured;
        phi_start = phi_measured;
        dphi_start = dphi_measured;
    end
    if start %|| (t_system - t_start) > 0.030
        t_start = t_system;
        l_start = l_measured;
        dl_start = dl_measured;
        phi_start = phi_measured;
        dphi_start = dphi_measured;
    end
    
    t = t_system - t_start;
    time_to_apex = t_apex - t_start;
    t = min(time_to_apex, t);

    % Virtual Leg Length
    [a0, a1, a2, a3] = ThirdOrderTrajectory(l_start, dl_start, l_apex, dl_apex, time_to_apex);
    l = a3*t^3 + a2*t^2 + a1*t + a0;
    dl = 3*a3*t^2 + 2*a2*t + a1;
    ddl = 6*a3*t + 2*a2;
    
    % Virtual Leg Angle
    [a0, a1, a2, a3] = ThirdOrderTrajectory(phi_start, dphi_start, phi_apex, dphi_apex, time_to_apex);
    phi = a3*t^3 + a2*t^2 + a1*t + a0;
    dphi = 3*a3*t^2 + 2*a2*t + a1;
    ddphi = 6*a3*t + 2*a2;

end

== matlab function smm_with_grf_tilting_2d/Control/Behavior Control/Primary Leg Behavior/Running/Flight/Deadbeat Placement/Virtual Leg to Four Bar ==
  data: l_leg input; dl_leg input; ddl_leg input; phi input; dphi input; ddphi input; back output; dback output; ddback output; front output; dfront output; ddfront output
function [back, dback, ddback, front, dfront, ddfront] = VirtualLegToFourBar(l_leg, dl_leg, ddl_leg, phi, dphi, ddphi)   
    [back, dback, ddback, front, dfront, ddfront] = VirtualLegToFourBar(l_leg, dl_leg, ddl_leg, phi, dphi, ddphi);
end

== matlab function smm_with_grf_tilting_2d/Control/Behavior Control/State Estimation/Kalman Filtering/Measurement Noise Covariance Matricies ==
  data: R_transverse output; vertical_GRF_L input; vertical_GRF_R input; R_kalman_foot_stance parameter; R_kalman_foot_slip parameter; R_kalman_dfoot_stance parameter; R_kalman_dfoot_slip parameter; sample_time parameter; m_total_real parameter; g parameter; R_vertical output; kalman_stance_slip_threshold parameter
function [R_transverse, R_vertical] =...
         MeasurementNoiseCovariance(vertical_GRF_L, vertical_GRF_R, ...
           R_kalman_foot_stance, R_kalman_foot_slip, R_kalman_dfoot_stance, R_kalman_dfoot_slip, sample_time, m_total_real, g, kalman_stance_slip_threshold)

    % filter states: [dx_w]; [dy_w]; [dz_w];
    % measurements:  [dx_w-dfL + dfL_hat; dx_w-dfR + dfR_hat]; 

    ratio_L = max(0, min(vertical_GRF_L/(kalman_stance_slip_threshold*m_total_real*g),1)); % ratio is 0 if no load, 1 if at least equilibrium
    ratio_R = max(0, min(vertical_GRF_R/(kalman_stance_slip_threshold*m_total_real*g),1));
    R_transverse = diag([ratio_L*R_kalman_dfoot_stance + (1-ratio_L)*R_kalman_dfoot_slip, ...
                         ratio_R*R_kalman_dfoot_stance + (1-ratio_R)*R_kalman_dfoot_slip])/sample_time;
    R_vertical = diag([ratio_L*R_kalman_foot_stance  + (1-ratio_L)*R_kalman_foot_slip,...
                       ratio_L*R_kalman_dfoot_stance + (1-ratio_L)*R_kalman_dfoot_slip,...
                       ratio_R*R_kalman_foot_stance  + (1-ratio_R)*R_kalman_foot_slip,...
                       ratio_R*R_kalman_dfoot_stance + (1-ratio_R)*R_kalman_dfoot_slip])/sample_time;
end
